simulink model "cyberAttack"  (R2022b)
settings: Solver=VariableStepAuto  StartTime=0.0  StopTime=10  RelTol=1e-3
values from neighbouring files (symbols this model uses):
  attackTimeDelay = 0.1    [editor.m]
  CC_Kd = 0    [editor.m]
  CC_Ki = 150    [editor.m]
  CC_Kp = 0    [editor.m]
  enableObserver = 1    [editor.m]
  ICapacity_1 = 3    [editor.m]
  ICapacity_2 = 2    [editor.m]
  ILoadFinal = 2    [editor.m]
  ILoadInitial = 3    [editor.m]
  Kd = 4.6e-4    (= 0.00046)    [editor.m]
  Ki = 6.15    [editor.m]
  Kp = 0.1    [editor.m]
  N = 2.56e3    (= 2560)    [editor.m]
  Rij = 0.05    [editor.m]
  Rt = 0.2    [editor.m]
  timeOfAttack = 5    [editor.m]
  tLoadChange = 6    [editor.m]
  Ts = 5e-5    (= 5e-05)    [editor.m]
  Vref = 40    [editor.m]
undefined symbols (not defined in the file or in its folder): Discrete, Time
libraries: fl_lib x27, nesl_utility_internal x15, slpidlib x4, simulink x2, ctrlSharedLib x2, ee_lib x2
(part 1 of 2)
settings Model: Creator=The MathWorks, Inc.  LastModifiedBy=bhuva

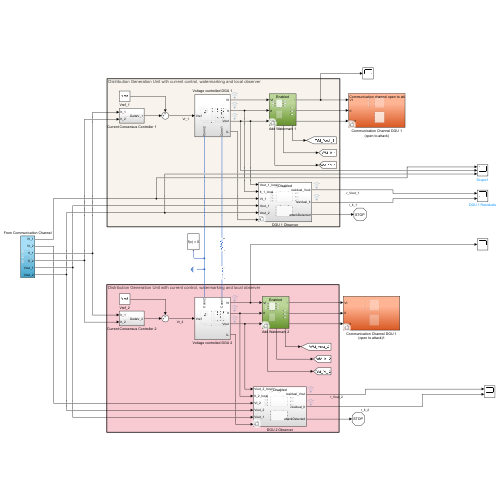
[thumbnail: Simulink's stored preview of the top-level diagram]
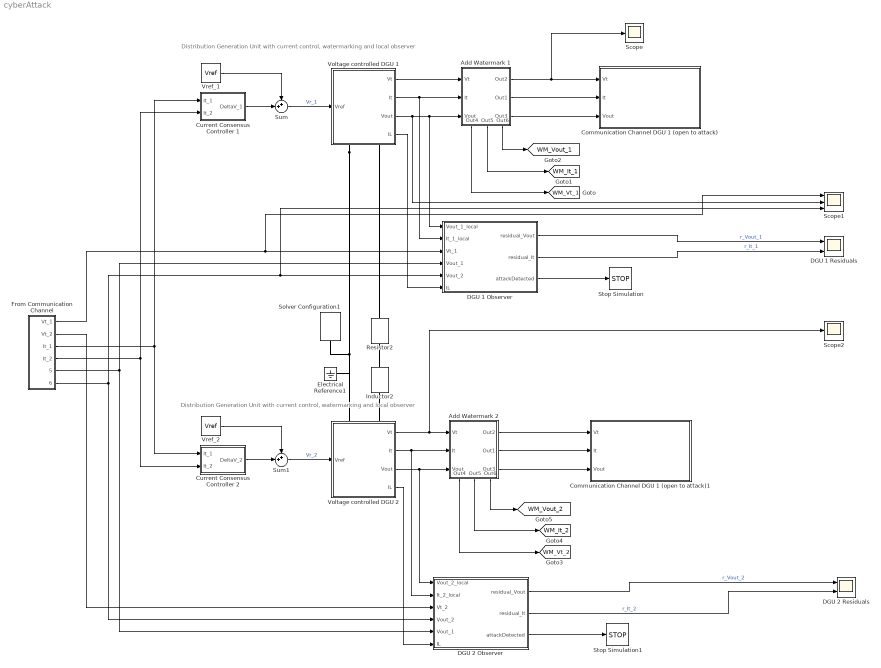
== system cyberAttack ==
  note: Distribution Generation Unit with current control, watermarking and local observer
  note: Distribution Generation Unit with current control, watermarking and local observer
  Add Watermark 1 : Subsystem  Variant=on  VariantControl=Choice
      settings: PortSchema="{\"entries\":[{\"content\":{\"sides\":[{\"content\":{\"connectorIds\":[\"In1\",\"In2\",\"In3\"]},\"type\":\"ConnectorPlacement.EquallySpacedRectSide\",\"uuid\":\"c94a7d77-0f2a-42c7-994c-f83d9f400b4a\"},{\"content\":{\"connectorIds\":[\"Out1\",\"Out2\",\"Out3\"],\"side\":\"RIGHT\"},\"type\":\"ConnectorPlacement.EquallySpacedRectSide\",\"uuid\":\"048bc904-366c-4deb-8d29-669922896a60\"},{\"content\":{\"connectorIds\":[],\"side\":\"TOP\"},\"type\":\"ConnectorPlacement.EquallySpacedRectSide\",\"uuid\":\"61856036-23df-49fc-9d48-72a95ac409b8\"},{\"content\":{\"connectorIds\":[\"Out4\",\"Out5\",\"Out6\"],\"side\":\"BOTTOM\"},\"type\":\"ConnectorPlacement.EquallySpacedRectSide\",\"uuid\":\"3c7882a6-545f-411e-a24e-2351be560f5c\"}]},\"type\":\"ConnectorPlacement.EquallySpacedConnector\",\"uuid\":\"82f313fb-6359-4167-9a1a-67611747de0f\"}],\"packageUris\":[\"http://schema.mathworks.com/mf0/Connector/R2020b\"],\"version\":\"1.0\"}"
  Add Watermark 2 : Subsystem  Variant=on  VariantControl=Choice
      settings: PortSchema="{\"entries\":[{\"content\":{\"sides\":[{\"content\":{\"connectorIds\":[\"In1\",\"In2\",\"In3\"]},\"type\":\"ConnectorPlacement.EquallySpacedRectSide\",\"uuid\":\"c94a7d77-0f2a-42c7-994c-f83d9f400b4a\"},{\"content\":{\"connectorIds\":[\"Out1\",\"Out2\",\"Out3\"],\"side\":\"RIGHT\"},\"type\":\"ConnectorPlacement.EquallySpacedRectSide\",\"uuid\":\"048bc904-366c-4deb-8d29-669922896a60\"},{\"content\":{\"connectorIds\":[],\"side\":\"TOP\"},\"type\":\"ConnectorPlacement.EquallySpacedRectSide\",\"uuid\":\"61856036-23df-49fc-9d48-72a95ac409b8\"},{\"content\":{\"connectorIds\":[\"Out4\",\"Out5\",\"Out6\"],\"side\":\"BOTTOM\"},\"type\":\"ConnectorPlacement.EquallySpacedRectSide\",\"uuid\":\"3c7882a6-545f-411e-a24e-2351be560f5c\"}]},\"type\":\"ConnectorPlacement.EquallySpacedConnector\",\"uuid\":\"82f313fb-6359-4167-9a1a-67611747de0f\"}],\"packageUris\":[\"http://schema.mathworks.com/mf0/Connector/R2020b\"],\"version\":\"1.0\"}"
  Communication Channel DGU 1 (open to attack) : Subsystem  Variant=on  VariantControl=Choice
  Communication Channel DGU 1 (open to attack)1 : Subsystem  Variant=on  VariantControl=Choice
  Current Consensus Controller 1 : Subsystem
  Current Consensus Controller 2 : Subsystem
  DGU 1 Observer : Subsystem  Variant=on  VariantControl=Choice
  DGU 1 Residuals : Scope  NumInputPorts=2
  DGU 2 Observer : Subsystem  Variant=on  VariantControl=Choice
  DGU 2 Residuals : Scope  NumInputPorts=2
  Electrical Reference1 : fl_lib/Electrical/Electrical Elements/Electrical Reference
  From Communication Channel : Subsystem
  Inductor2 : fl_lib/Electrical/Electrical Elements/Inductor  l=Lij H  r=0 Ohm  g=1e-9 1/Ohm  i_specify=off  i_priority=None  i=0 A  i_nominal_specify=off  i_nominal_unit=A  i_nominal_value=1  v_specify=off  v_priority=None  v=0 V  v_nominal_specify=off  v_nominal_unit=V  v_nominal_value=1  i_L_specify=off  i_L_priority=High  i_L=0 A  i_L_nominal_specify=off  i_L_nominal_unit=A  i_L_nominal_value=1
  Resistor2 : fl_lib/Electrical/Electrical Elements/Resistor  R=Rij Ohm  i_specify=off  i_priority=None  i=0 A  i_nominal_specify=off  i_nominal_unit=A  i_nominal_value=1  v_specify=off  v_priority=None  v=0 V  v_nominal_specify=off  v_nominal_unit=V  v_nominal_value=1
  Scope : Scope
  Scope1 : Scope  NumInputPorts=3
  Scope2 : Scope
  Solver Configuration1 : nesl_utility_internal/Solver Configuration  PhysicalDomain=network_engine_domain  SubClassName=solver  LeftPortType=input  RightPortType=generic  Tones=[]  Harmonics=[]  SimulateNoise=off  Profile=off  UseLocalSampling=off  EnableSwitchedLinearOptims=on  FrequencyDomain=off  UseCCode=off  RelTol=0.001  AbsTol=1e-06  MinStep=1e-09  ToWorkspace=off  RevertToSquareIcSolve=off  NumHomotopyIterations=100  PhasorMode=off  PhasorModeNumHarmonics=1  ConsistencySolver=NEWTON_FTOL  IndexReductionMethod=DerivativeReplacement  DoDC=off  ResidualTolerance=1e-9  ConsistencyTolSource=GLOBAL  ConsistencyAbsTol=0.001  ConsistencyRelTol=0.001  ConsistencyTolFactor=0.001  UseLocalSolver=on  LocalSolverChoice=NE_BACKWARD_EULER_ADVANCER  ResolveIndetEquations=on  FunctionEvalNumThread=1  LocalSolverSampleTime=Ts  DoFixedCost=on  MaxNonlinIter=3  MaxModeIter=2  ComputeImpulses=off  ImpulseIterations=2  LinearAlgebra=auto  LinearAlgebraNumThread=0  EquationFormulation=NE_TIME_EF  DelaysMemoryBudget=1024  AutomaticFiltering=on  FilteringTimeConstant=0.001  PartitionStorageMethod=AS_NEEDED  PartitionMemoryBudget=1024  PartitionMethod=FAST
  Stop Simulation : Stop
  Stop Simulation1 : Stop
  Sum : Sum  Inputs=++|
  Sum1 : Sum  Inputs=++|
  Voltage controlled DGU 1 : Subsystem
      settings: PortSchema="{\"entries\":[{\"content\":{\"sides\":[{\"content\":{\"connectorIds\":[]},\"type\":\"ConnectorPlacement.EquallySpacedRectSide\",\"uuid\":\"bd1f37b5-cace-475a-9319-df5dc175988c\"},{\"content\":{\"connectorIds\":[\"RConn1\",\"RConn2\"],\"side\":\"RIGHT\"},\"type\":\"ConnectorPlacement.EquallySpacedRectSide\",\"uuid\":\"6e9492d2-b492-4ddc-9bf9-c37fa50387fb\"},{\"content\":{\"connectorIds\":[\"Out1\",\"Out2\",\"Out3\",\"Out4\"],\"side\":\"TOP\"},\"type\":\"ConnectorPlacement.EquallySpacedRectSide\",\"uuid\":\"740d822e-a5fc-4d01-8f2e-7dd9c8c34700\"},{\"content\":{\"connectorIds\":[\"In1\"],\"side\":\"BOTTOM\"},\"type\":\"ConnectorPlacement.EquallySpacedRectSide\",\"uuid\":\"ce7350ec-18c7-472a-9669-30fb5abf65bf\"}]},\"type\":\"ConnectorPlacement.EquallySpacedConnector\",\"uuid\":\"15ef9329-fda5-41fa-bf9c-9b9fdaa2cf39\"}],\"packageUris\":[\"http://schema.mathworks.com/mf0/Connector/R2020b\"],\"version\":\"1.0\"}"
  Voltage controlled DGU 2 : Subsystem
      settings: PortSchema="{\"entries\":[{\"content\":{\"sides\":[{\"content\":{\"connectorIds\":[]},\"type\":\"ConnectorPlacement.EquallySpacedRectSide\",\"uuid\":\"bd1f37b5-cace-475a-9319-df5dc175988c\"},{\"content\":{\"connectorIds\":[\"RConn1\",\"RConn2\"],\"side\":\"RIGHT\"},\"type\":\"ConnectorPlacement.EquallySpacedRectSide\",\"uuid\":\"6e9492d2-b492-4ddc-9bf9-c37fa50387fb\"},{\"content\":{\"connectorIds\":[\"Out1\",\"Out2\",\"Out3\",\"Out4\"],\"side\":\"TOP\"},\"type\":\"ConnectorPlacement.EquallySpacedRectSide\",\"uuid\":\"740d822e-a5fc-4d01-8f2e-7dd9c8c34700\"},{\"content\":{\"connectorIds\":[\"In1\"],\"side\":\"BOTTOM\"},\"type\":\"ConnectorPlacement.EquallySpacedRectSide\",\"uuid\":\"ce7350ec-18c7-472a-9669-30fb5abf65bf\"}]},\"type\":\"ConnectorPlacement.EquallySpacedConnector\",\"uuid\":\"15ef9329-fda5-41fa-bf9c-9b9fdaa2cf39\"}],\"packageUris\":[\"http://schema.mathworks.com/mf0/Connector/R2020b\"],\"version\":\"1.0\"}"
  Vref_1 : Constant  Value=Vref  SampleTime=Ts
  Vref_2 : Constant  Value=Vref  SampleTime=Ts
  tag scope: WM_It_1=global, WM_It_2=global, WM_Vout_1=global, WM_Vout_2=global, WM_Vt_1=global, WM_Vt_2=global
  wires:
  Vref_1/1 -> Sum/1
  Sum/1 -> Voltage controlled DGU 1/1(Vref)  "Vr_1"
  Current Consensus Controller 1/1(DeltaV_1) -> Sum/2
  From Communication Channel/4(It_2) -> Current Consensus Controller 1/2(It_2), Current Consensus Controller 2/2(It_2)
  Voltage controlled DGU 1/3(Vout) -> Scope1/2, Add Watermark 1/3(Vout), DGU 1 Observer/1(Vout_1_local)
  Current Consensus Controller 2/1(DeltaV_2) -> Sum1/2
  Voltage controlled DGU 2/3(It) -> Add Watermark 2/2(It), DGU 2 Observer/2(It_2_local)
  Voltage controlled DGU 2/4(Vt) -> Scope2/1, Add Watermark 2/1(Vt)
  From Communication Channel/3(It_1) -> Current Consensus Controller 1/1(It_1), Current Consensus Controller 2/1(It_1)
  From Communication Channel/6(Vout_2) -> DGU 2 Observer/4(Vout_2), Scope1/3, DGU 1 Observer/5(Vout_2)
  Sum1/1 -> Voltage controlled DGU 2/1(Vref)  "Vr_2"
  From Communication Channel/5(Vout_1) -> DGU 2 Observer/5(Vout_1), DGU 1 Observer/4(Vout_1)
  Voltage controlled DGU 2/2(Vout) -> Add Watermark 2/3(Vout), DGU 2 Observer/1(Vout_2_local)
  Vref_2/1 -> Sum1/1
  Voltage controlled DGU 1/2(It) -> Add Watermark 1/2(It), DGU 1 Observer/2(It_1_local)
  DGU 2 Observer/3(attackDetected) -> Stop Simulation1/1
  From Communication Channel/1(Vt_1) -> Scope1/1, DGU 1 Observer/3(Vt_1)
  Voltage controlled DGU 1/4(IL) -> DGU 1 Observer/6(IL)
  From Communication Channel/2(Vt_2) -> DGU 2 Observer/3(Vt_2)
  Voltage controlled DGU 1/1(Vt) -> Add Watermark 1/1(Vt)
  Add Watermark 1/1(Out2) -> Scope/1, Communication Channel DGU 1 (open to attack)/1(Vt)
  Add Watermark 1/2(Out1) -> Communication Channel DGU 1 (open to attack)/2(It)
  Add Watermark 1/3(Out3) -> Communication Channel DGU 1 (open to attack)/3(Vout)
  Add Watermark 1/4(Out4) -> [WM_Vt_1]
  Add Watermark 1/5(Out5) -> [WM_It_1]
  Add Watermark 1/6(Out6) -> [WM_Vout_1]
  DGU 1 Observer/1(residual_Vout) -> DGU 1 Residuals/1  "r_Vout_1"
  DGU 1 Observer/2(residual_It) -> DGU 1 Residuals/2  "r_It_1"
  DGU 1 Observer/3(attackDetected) -> Stop Simulation/1
  Voltage controlled DGU 2/1(IL) -> DGU 2 Observer/6(IL)
  DGU 2 Observer/1(residual_Vout) -> DGU 2 Residuals/1  "r_Vout_2"
  DGU 2 Observer/2(residual_It) -> DGU 2 Residuals/2  "r_It_2"
  Add Watermark 2/6(Out6) -> [WM_Vout_2]
  Add Watermark 2/5(Out5) -> [WM_It_2]
  Add Watermark 2/4(Out4) -> [WM_Vt_2]
  Add Watermark 2/1(Out2) -> Communication Channel DGU 1 (open to attack)1/1(Vt)
  Add Watermark 2/2(Out1) -> Communication Channel DGU 1 (open to attack)1/2(It)
  Add Watermark 2/3(Out3) -> Communication Channel DGU 1 (open to attack)1/3(Vout)
  connections:
  Voltage controlled DGU 1/RConn2 -- Electrical Reference1/LConn1 -- Voltage controlled DGU 2/RConn2 -- Solver Configuration1/RConn1
  Inductor2/LConn1 -- Resistor2/RConn1
  Voltage controlled DGU 2/RConn1 -- Inductor2/RConn1
  Resistor2/LConn1 -- Voltage controlled DGU 1/RConn1

== system cyberAttack/Add Watermark 1 ==
  Vt : Inport
  It : Inport  Port=2
  Vout : Inport  Port=3
  Disabled : Subsystem  VariantControl=enableWatermarking == 0
      settings: PortSchema="{\"entries\":[{\"content\":{\"sides\":[{\"content\":{\"connectorIds\":[\"In1\",\"In2\",\"In3\"]},\"type\":\"ConnectorPlacement.EquallySpacedRectSide\",\"uuid\":\"c94a7d77-0f2a-42c7-994c-f83d9f400b4a\"},{\"content\":{\"connectorIds\":[\"Out1\",\"Out2\",\"Out3\"],\"side\":\"RIGHT\"},\"type\":\"ConnectorPlacement.EquallySpacedRectSide\",\"uuid\":\"048bc904-366c-4deb-8d29-669922896a60\"},{\"content\":{\"connectorIds\":[],\"side\":\"TOP\"},\"type\":\"ConnectorPlacement.EquallySpacedRectSide\",\"uuid\":\"61856036-23df-49fc-9d48-72a95ac409b8\"},{\"content\":{\"connectorIds\":[\"Out4\",\"Out5\",\"Out6\"],\"side\":\"BOTTOM\"},\"type\":\"ConnectorPlacement.EquallySpacedRectSide\",\"uuid\":\"3c7882a6-545f-411e-a24e-2351be560f5c\"}]},\"type\":\"ConnectorPlacement.EquallySpacedConnector\",\"uuid\":\"82f313fb-6359-4167-9a1a-67611747de0f\"}],\"packageUris\":[\"http://schema.mathworks.com/mf0/Connector/R2020b\"],\"version\":\"1.0\"}"
  Enabled : Subsystem  VariantControl=enableWatermarking == 1
      settings: PortSchema="{\"entries\":[{\"content\":{\"sides\":[{\"content\":{\"connectorIds\":[\"In1\",\"In2\",\"In3\"]},\"type\":\"ConnectorPlacement.EquallySpacedRectSide\",\"uuid\":\"c94a7d77-0f2a-42c7-994c-f83d9f400b4a\"},{\"content\":{\"connectorIds\":[\"Out1\",\"Out2\",\"Out3\"],\"side\":\"RIGHT\"},\"type\":\"ConnectorPlacement.EquallySpacedRectSide\",\"uuid\":\"048bc904-366c-4deb-8d29-669922896a60\"},{\"content\":{\"connectorIds\":[],\"side\":\"TOP\"},\"type\":\"ConnectorPlacement.EquallySpacedRectSide\",\"uuid\":\"61856036-23df-49fc-9d48-72a95ac409b8\"},{\"content\":{\"connectorIds\":[\"Out4\",\"Out5\",\"Out6\"],\"side\":\"BOTTOM\"},\"type\":\"ConnectorPlacement.EquallySpacedRectSide\",\"uuid\":\"3c7882a6-545f-411e-a24e-2351be560f5c\"}]},\"type\":\"ConnectorPlacement.EquallySpacedConnector\",\"uuid\":\"82f313fb-6359-4167-9a1a-67611747de0f\"}],\"packageUris\":[\"http://schema.mathworks.com/mf0/Connector/R2020b\"],\"version\":\"1.0\"}"
  Out2 : Outport
  Out1 : Outport  Port=2
  Out3 : Outport  Port=3
  Out4 : Outport  Port=4
  Out5 : Outport  Port=5
  Out6 : Outport  Port=6

== system cyberAttack/Add Watermark 2 ==
  Vt : Inport
  It : Inport  Port=2
  Vout : Inport  Port=3
  Disabled : Subsystem  VariantControl=enableWatermarking == 0
      settings: PortSchema="{\"entries\":[{\"content\":{\"sides\":[{\"content\":{\"connectorIds\":[\"In1\",\"In2\",\"In3\"]},\"type\":\"ConnectorPlacement.EquallySpacedRectSide\",\"uuid\":\"c94a7d77-0f2a-42c7-994c-f83d9f400b4a\"},{\"content\":{\"connectorIds\":[\"Out1\",\"Out2\",\"Out3\"],\"side\":\"RIGHT\"},\"type\":\"ConnectorPlacement.EquallySpacedRectSide\",\"uuid\":\"048bc904-366c-4deb-8d29-669922896a60\"},{\"content\":{\"connectorIds\":[],\"side\":\"TOP\"},\"type\":\"ConnectorPlacement.EquallySpacedRectSide\",\"uuid\":\"61856036-23df-49fc-9d48-72a95ac409b8\"},{\"content\":{\"connectorIds\":[\"Out4\",\"Out5\",\"Out6\"],\"side\":\"BOTTOM\"},\"type\":\"ConnectorPlacement.EquallySpacedRectSide\",\"uuid\":\"3c7882a6-545f-411e-a24e-2351be560f5c\"}]},\"type\":\"ConnectorPlacement.EquallySpacedConnector\",\"uuid\":\"82f313fb-6359-4167-9a1a-67611747de0f\"}],\"packageUris\":[\"http://schema.mathworks.com/mf0/Connector/R2020b\"],\"version\":\"1.0\"}"
  Enabled : Subsystem  VariantControl=enableWatermarking == 1
      settings: PortSchema="{\"entries\":[{\"content\":{\"sides\":[{\"content\":{\"connectorIds\":[\"In1\",\"In2\",\"In3\"]},\"type\":\"ConnectorPlacement.EquallySpacedRectSide\",\"uuid\":\"c94a7d77-0f2a-42c7-994c-f83d9f400b4a\"},{\"content\":{\"connectorIds\":[\"Out1\",\"Out2\",\"Out3\"],\"side\":\"RIGHT\"},\"type\":\"ConnectorPlacement.EquallySpacedRectSide\",\"uuid\":\"048bc904-366c-4deb-8d29-669922896a60\"},{\"content\":{\"connectorIds\":[],\"side\":\"TOP\"},\"type\":\"ConnectorPlacement.EquallySpacedRectSide\",\"uuid\":\"61856036-23df-49fc-9d48-72a95ac409b8\"},{\"content\":{\"connectorIds\":[\"Out4\",\"Out5\",\"Out6\"],\"side\":\"BOTTOM\"},\"type\":\"ConnectorPlacement.EquallySpacedRectSide\",\"uuid\":\"3c7882a6-545f-411e-a24e-2351be560f5c\"}]},\"type\":\"ConnectorPlacement.EquallySpacedConnector\",\"uuid\":\"82f313fb-6359-4167-9a1a-67611747de0f\"}],\"packageUris\":[\"http://schema.mathworks.com/mf0/Connector/R2020b\"],\"version\":\"1.0\"}"
  Out2 : Outport
  Out1 : Outport  Port=2
  Out3 : Outport  Port=3
  Out4 : Outport  Port=4
  Out5 : Outport  Port=5
  Out6 : Outport  Port=6

== system cyberAttack/Communication Channel DGU 1 (open to attack) ==
  Vt : Inport
  It : Inport  Port=2
  Vout : Inport  Port=3
  Communication Channel : Subsystem  VariantControl=enableAttack == 0
  Communication channel open to attack : Subsystem  VariantControl=enableAttack == 1

== system cyberAttack/Communication Channel DGU 1 (open to attack)1 ==
  Vt : Inport
  It : Inport  Port=2
  Vout : Inport  Port=3
  Communication Channel : Subsystem  VariantControl=enableAttack1 == 0
  Communication channel open to attack : Subsystem  VariantControl=enableAttack1 == 1

== system cyberAttack/Current Consensus Controller 1 ==
  It_1 : Inport
  It_2 : Inport  Port=2
  Discrete PID Controller : slpidlib/PID Controller  Controller=PID  Form=Parallel  TimeDomain=Discrete-time  UseExternalTs=off  SampleTime=Ts  IntegratorMethod=Forward Euler  FilterMethod=Forward Euler  ControllerParametersSource=internal  P=CC_Kp  I=CC_Ki  UseKiTs=off  D=CC_Kd  N=1e4  UseFilter=on  TunerSelectOption=Transfer Function Based (PID Tuner App)  InitialConditionSource=internal  InitialConditionForIntegrator=0  InitialConditionForFilter=0  DifferentiatorICPrevScaledInput=0  ExternalReset=none  TrackingMode=off  Kt=1  LimitOutput=off  SatLimitsSource=internal  UpperSaturationLimit=inf  LowerSaturationLimit=-inf  LinearizeAsGain=off  AntiWindupMode=none  Kb=1  LimitIntegrator=off  UpperIntegratorSaturationLimit=inf  LowerIntegratorSaturationLimit=-inf  POutMin=[]  POutMax=[]  IOutMin=[]  IOutMax=[]  DOutMin=[]  DOutMax=[]  NOutMin=[]  NOutMax=[]  SumOutMin=[]  SumOutMax=[]  SaturationOutMin=[]  SaturationOutMax=[]  PParamMin=[]  PParamMax=[]  IParamMin=[]  IParamMax=[]  DParamMin=[]  DParamMax=[]  NParamMin=[]  NParamMax=[]  KbParamMin=[]  KbParamMax=[]  KtParamMin=[]  KtParamMax=[]  KbOutMin=[]  KbOutMax=[]  KtOutMin=[]  KtOutMax=[]  IntegratorOutMin=[]  IntegratorOutMax=[]  FilterOutMin=[]  FilterOutMax=[]  SumI1OutMin=[]  SumI1OutMax=[]  SumI2OutMin=[]  SumI2OutMax=[]  SumI3OutMin=[]  SumI3OutMax=[]  SumI4OutMin=[]  SumI4OutMax=[]  SumDOutMin=[]  SumDOutMax=[]  DifferentiatorOutMin=[]  DifferentiatorOutMax=[]  FilterDiffOutCoefMin=[]  FilterDiffOutCoefMax=[]  ReciprocalOutMin=[]  ReciprocalOutMax=[]  SumDenOutMin=[]  SumDenOutMax=[]  SumNumOutMin=[]  SumNumOutMax=[]  DivideOutMin=[]  DivideOutMax=[]  UdiffTsProdOutMin=[]  UdiffTsProdOutMax=[]  NTsProdOutMin=[]  NTsProdOutMax=[]  UintegralTsProdOutMin=[]  UintegralTsProdOutMax=[]  UngainTsProdOutMin=[]  UngainTsProdOutMax=[]  ClampingZeroOutDataTypeStr=Inherit: Inherit via back propagation  ClampingZeroOutMin=[]  ClampingZeroOutMax=[]  FilterDenConstantOutDataTypeStr=Inherit: Inherit via back propagation  FilterDenConstantOutMin=[]  FilterDenConstantOutMax=[]  PCopyOutDataTypeStr=Inherit: Inherit via back propagation  PCopyOutMin=[]  PCopyOutMax=[]  NCopyOutDataTypeStr=Inherit: Inherit via back propagation  NCopyOutMin=[]  NCopyOutMax=[]  IntegratorContinuousStateAttributes=''  IntegratorStateMustResolveToSignalObject=off  IntegratorRTWStateStorageClass=Auto  FilterContinuousStateAttributes=''  FilterStateMustResolveToSignalObject=off  FilterRTWStateStorageClass=Auto  ParallelPVariant=InternalParameters  IdealPVariant=Disabled  IVariant=InternalParameters  DVariant=InternalParameters  IntegratorVariant=Discrete  SatVariant=Disabled  AWVariant=Passthrough  PCopyVariant=Disabled  TRVariant=Disabled  FdbkBlocksVariant=Forward  IdealPFdbkVariant=Disabled  SatFdbkVariant=Disabled  DerivativeFilterVariant=ForwardEulerFilter  NVariant=InternalParameters  NCopyVariant=Disabled  FilterICVariant=InternalICsFilter  IntegratorICVariant=InternalICs  ExternalResetVariant=Disabled  TRSumVariant=Passthrough  SumFdbkVariant=Disabled  SumVariant=Sum_PID  TsampFilterVariant=InternalTs  TsampNgainVariant=Passthrough  TsampIntegralVariant=Passthrough  ExternalSaturationOutDataTypeStr=Inherit: Same as second input
      settings: LibrarySourceBlock=simulink/Discrete/Discrete PID Controller
  Gain7 : Gain  Gain=1/ICapacity_1
  Gain8 : Gain  Gain=1/ICapacity_2
  Sum : Sum  Inputs=-+|
  Sum1 : Sum  Inputs=-+|
  Sum4 : Sum  Inputs=|-+
  DeltaV_1 : Outport
  wires:
  Gain8/1 -> Sum4/2
  It_2/1 -> Sum1/2
  Gain7/1 -> Sum4/1
  Discrete PID Controller/1 -> DeltaV_1/1
  Sum/1 -> Gain7/1
  Sum1/1 -> Gain8/1
  It_1/1 -> Sum/2
  [WM_It_1] -> Sum/1
  [WM_It_2] -> Sum1/1
  Sum4/1 -> Discrete PID Controller/1

== system cyberAttack/Current Consensus Controller 2 ==
  It_1 : Inport
  It_2 : Inport  Port=2
  Discrete PID Controller : slpidlib/PID Controller  Controller=PID  Form=Parallel  TimeDomain=Discrete-time  UseExternalTs=off  SampleTime=Ts  IntegratorMethod=Forward Euler  FilterMethod=Forward Euler  ControllerParametersSource=internal  P=CC_Kp  I=CC_Ki  UseKiTs=off  D=CC_Kd  N=1e4  UseFilter=on  TunerSelectOption=Transfer Function Based (PID Tuner App)  InitialConditionSource=internal  InitialConditionForIntegrator=0  InitialConditionForFilter=0  DifferentiatorICPrevScaledInput=0  ExternalReset=none  TrackingMode=off  Kt=1  LimitOutput=off  SatLimitsSource=internal  UpperSaturationLimit=inf  LowerSaturationLimit=-inf  LinearizeAsGain=off  AntiWindupMode=none  Kb=1  LimitIntegrator=off  UpperIntegratorSaturationLimit=inf  LowerIntegratorSaturationLimit=-inf  POutMin=[]  POutMax=[]  IOutMin=[]  IOutMax=[]  DOutMin=[]  DOutMax=[]  NOutMin=[]  NOutMax=[]  SumOutMin=[]  SumOutMax=[]  SaturationOutMin=[]  SaturationOutMax=[]  PParamMin=[]  PParamMax=[]  IParamMin=[]  IParamMax=[]  DParamMin=[]  DParamMax=[]  NParamMin=[]  NParamMax=[]  KbParamMin=[]  KbParamMax=[]  KtParamMin=[]  KtParamMax=[]  KbOutMin=[]  KbOutMax=[]  KtOutMin=[]  KtOutMax=[]  IntegratorOutMin=[]  IntegratorOutMax=[]  FilterOutMin=[]  FilterOutMax=[]  SumI1OutMin=[]  SumI1OutMax=[]  SumI2OutMin=[]  SumI2OutMax=[]  SumI3OutMin=[]  SumI3OutMax=[]  SumI4OutMin=[]  SumI4OutMax=[]  SumDOutMin=[]  SumDOutMax=[]  DifferentiatorOutMin=[]  DifferentiatorOutMax=[]  FilterDiffOutCoefMin=[]  FilterDiffOutCoefMax=[]  ReciprocalOutMin=[]  ReciprocalOutMax=[]  SumDenOutMin=[]  SumDenOutMax=[]  SumNumOutMin=[]  SumNumOutMax=[]  DivideOutMin=[]  DivideOutMax=[]  UdiffTsProdOutMin=[]  UdiffTsProdOutMax=[]  NTsProdOutMin=[]  NTsProdOutMax=[]  UintegralTsProdOutMin=[]  UintegralTsProdOutMax=[]  UngainTsProdOutMin=[]  UngainTsProdOutMax=[]  ClampingZeroOutDataTypeStr=Inherit: Inherit via back propagation  ClampingZeroOutMin=[]  ClampingZeroOutMax=[]  FilterDenConstantOutDataTypeStr=Inherit: Inherit via back propagation  FilterDenConstantOutMin=[]  FilterDenConstantOutMax=[]  PCopyOutDataTypeStr=Inherit: Inherit via back propagation  PCopyOutMin=[]  PCopyOutMax=[]  NCopyOutDataTypeStr=Inherit: Inherit via back propagation  NCopyOutMin=[]  NCopyOutMax=[]  IntegratorContinuousStateAttributes=''  IntegratorStateMustResolveToSignalObject=off  IntegratorRTWStateStorageClass=Auto  FilterContinuousStateAttributes=''  FilterStateMustResolveToSignalObject=off  FilterRTWStateStorageClass=Auto  ParallelPVariant=InternalParameters  IdealPVariant=Disabled  IVariant=InternalParameters  DVariant=InternalParameters  IntegratorVariant=Discrete  SatVariant=Disabled  AWVariant=Passthrough  PCopyVariant=Disabled  TRVariant=Disabled  FdbkBlocksVariant=Forward  IdealPFdbkVariant=Disabled  SatFdbkVariant=Disabled  DerivativeFilterVariant=ForwardEulerFilter  NVariant=InternalParameters  NCopyVariant=Disabled  FilterICVariant=InternalICsFilter  IntegratorICVariant=InternalICs  ExternalResetVariant=Disabled  TRSumVariant=Passthrough  SumFdbkVariant=Disabled  SumVariant=Sum_PID  TsampFilterVariant=InternalTs  TsampNgainVariant=Passthrough  TsampIntegralVariant=Passthrough  ExternalSaturationOutDataTypeStr=Inherit: Same as second input
      settings: LibrarySourceBlock=simulink/Discrete/Discrete PID Controller
  Gain7 : Gain  Gain=1/ICapacity_1
  Gain8 : Gain  Gain=1/ICapacity_2
  Sum : Sum  Inputs=-+|
  Sum1 : Sum  Inputs=-+|
  Sum4 : Sum  Inputs=|+-
  DeltaV_2 : Outport
  wires:
  Gain8/1 -> Sum4/2
  It_2/1 -> Sum1/2
  Sum4/1 -> Discrete PID Controller/1
  Gain7/1 -> Sum4/1
  Discrete PID Controller/1 -> DeltaV_2/1
  Sum/1 -> Gain7/1
  Sum1/1 -> Gain8/1
  It_1/1 -> Sum/2
  [WM_It_1] -> Sum/1
  [WM_It_2] -> Sum1/1

== system cyberAttack/DGU 1 Observer ==
  Vout_1_local : Inport
  It_1_local : Inport  Port=2
  Vt_1 : Inport  Port=3
  Vout_1 : Inport  Port=4
  Vout_2 : Inport  Port=5
  IL : Inport  Port=6
  Disabled : Subsystem  VariantControl=enableObserver == 0
      settings: PortSchema="{\"entries\":[{\"content\":{\"sides\":[{\"content\":{\"connectorIds\":[\"In1\",\"In2\",\"In3\",\"In4\"]},\"type\":\"ConnectorPlacement.EquallySpacedRectSide\",\"uuid\":\"1fcbc3c4-c380-448d-a7a8-357aa057b5ad\"},{\"content\":{\"connectorIds\":[\"Out1\",\"Out2\",\"Out3\"],\"side\":\"RIGHT\"},\"type\":\"ConnectorPlacement.EquallySpacedRectSide\",\"uuid\":\"7cbaad62-7890-4094-8ace-3159eca04825\"},{\"content\":{\"connectorIds\":[\"In5\",\"In6\"],\"side\":\"TOP\"},\"type\":\"ConnectorPlacement.EquallySpacedRectSide\",\"uuid\":\"f6c34017-9df2-4479-96e0-d67eb53c1d2d\"}]},\"type\":\"ConnectorPlacement.EquallySpacedConnector\",\"uuid\":\"f0a4a9b8-ed06-4c65-915f-6b202d377626\"}],\"packageUris\":[\"http://schema.mathworks.com/mf0/Connector/R2020b\"],\"version\":\"1.0\"}"
  Enabled : Subsystem  VariantControl=enableObserver == 1
      settings: PortSchema="{\"entries\":[{\"content\":{\"sides\":[{\"content\":{\"connectorIds\":[\"In1\",\"In2\",\"In3\",\"In4\"]},\"type\":\"ConnectorPlacement.EquallySpacedRectSide\",\"uuid\":\"1fcbc3c4-c380-448d-a7a8-357aa057b5ad\"},{\"content\":{\"connectorIds\":[\"Out1\",\"Out2\",\"Out3\"],\"side\":\"RIGHT\"},\"type\":\"ConnectorPlacement.EquallySpacedRectSide\",\"uuid\":\"7cbaad62-7890-4094-8ace-3159eca04825\"},{\"content\":{\"connectorIds\":[\"In5\",\"In6\"],\"side\":\"TOP\"},\"type\":\"ConnectorPlacement.EquallySpacedRectSide\",\"uuid\":\"f6c34017-9df2-4479-96e0-d67eb53c1d2d\"}]},\"type\":\"ConnectorPlacement.EquallySpacedConnector\",\"uuid\":\"f0a4a9b8-ed06-4c65-915f-6b202d377626\"}],\"packageUris\":[\"http://schema.mathworks.com/mf0/Connector/R2020b\"],\"version\":\"1.0\"}"
  residual_Vout : Outport
  residual_It : Outport  Port=2
  attackDetected : Outport  Port=3

== system cyberAttack/DGU 2 Observer ==
  Vout_2_local : Inport
  It_2_local : Inport  Port=2
  Vt_2 : Inport  Port=3
  Vout_2 : Inport  Port=4
  Vout_1 : Inport  Port=5
  IL : Inport  Port=6
  Disabled : Subsystem  VariantControl=enableObserver == 0
      settings: PortSchema="{\"entries\":[{\"content\":{\"sides\":[{\"content\":{\"connectorIds\":[\"In1\",\"In2\",\"In3\",\"In4\"]},\"type\":\"ConnectorPlacement.EquallySpacedRectSide\",\"uuid\":\"1fcbc3c4-c380-448d-a7a8-357aa057b5ad\"},{\"content\":{\"connectorIds\":[\"Out1\",\"Out2\",\"Out3\"],\"side\":\"RIGHT\"},\"type\":\"ConnectorPlacement.EquallySpacedRectSide\",\"uuid\":\"7cbaad62-7890-4094-8ace-3159eca04825\"},{\"content\":{\"connectorIds\":[\"In5\",\"In6\"],\"side\":\"TOP\"},\"type\":\"ConnectorPlacement.EquallySpacedRectSide\",\"uuid\":\"f6c34017-9df2-4479-96e0-d67eb53c1d2d\"}]},\"type\":\"ConnectorPlacement.EquallySpacedConnector\",\"uuid\":\"f0a4a9b8-ed06-4c65-915f-6b202d377626\"}],\"packageUris\":[\"http://schema.mathworks.com/mf0/Connector/R2020b\"],\"version\":\"1.0\"}"
  Enabled : Subsystem  VariantControl=enableObserver == 1
      settings: PortSchema="{\"entries\":[{\"content\":{\"sides\":[{\"content\":{\"connectorIds\":[\"In1\",\"In2\",\"In3\",\"In4\"]},\"type\":\"ConnectorPlacement.EquallySpacedRectSide\",\"uuid\":\"1fcbc3c4-c380-448d-a7a8-357aa057b5ad\"},{\"content\":{\"connectorIds\":[\"Out1\",\"Out2\",\"Out3\"],\"side\":\"RIGHT\"},\"type\":\"ConnectorPlacement.EquallySpacedRectSide\",\"uuid\":\"7cbaad62-7890-4094-8ace-3159eca04825\"},{\"content\":{\"connectorIds\":[\"In5\",\"In6\"],\"side\":\"TOP\"},\"type\":\"ConnectorPlacement.EquallySpacedRectSide\",\"uuid\":\"f6c34017-9df2-4479-96e0-d67eb53c1d2d\"}]},\"type\":\"ConnectorPlacement.EquallySpacedConnector\",\"uuid\":\"f0a4a9b8-ed06-4c65-915f-6b202d377626\"}],\"packageUris\":[\"http://schema.mathworks.com/mf0/Connector/R2020b\"],\"version\":\"1.0\"}"
  residual_Vout : Outport
  residual_It : Outport  Port=2
  attackDetected : Outport  Port=3

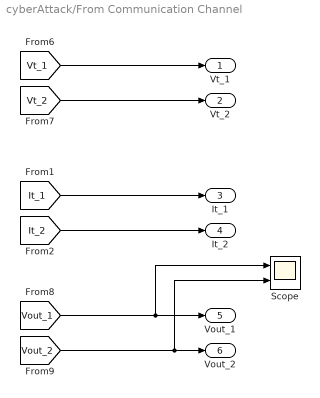
== system cyberAttack/From Communication Channel ==
  Scope : Scope  NumInputPorts=2
  Vt_1 : Outport
  Vt_2 : Outport  Port=2
  It_1 : Outport  Port=3
  It_2 : Outport  Port=4
  Vout_1 : Outport  Port=5
  Vout_2 : Outport  Port=6
  wires:
  [Vout_2] -> Scope/2, Vout_2/1
  [Vt_1] -> Vt_1/1
  [It_1] -> It_1/1
  [Vout_1] -> Scope/1, Vout_1/1
  [Vt_2] -> Vt_2/1
  [It_2] -> It_2/1

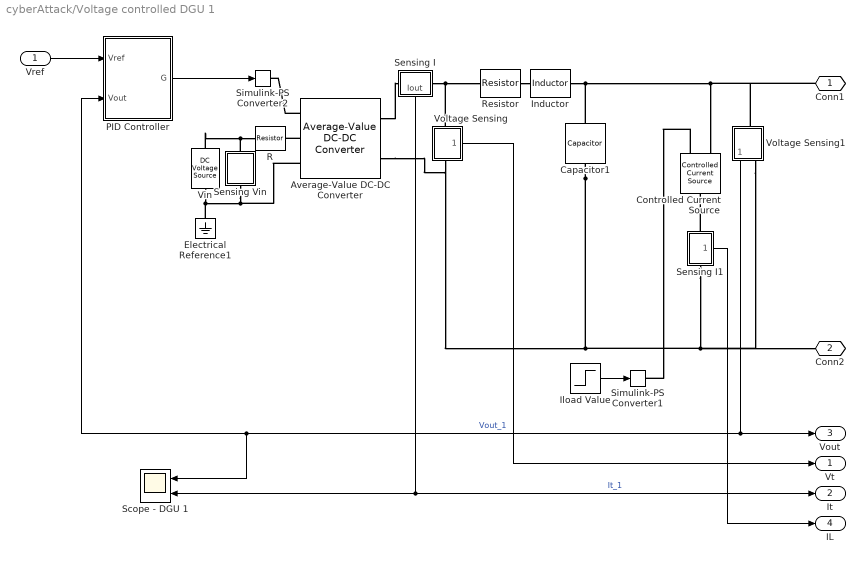
== system cyberAttack/Voltage controlled DGU 1 ==
  Vref : Inport
  Average-Value DC-DC Converter : ee_lib/Semiconductors & Converters/Converters/Average-Value DC-DC Converter  control_option=ee.enum.converters.controlinput.dutycycle  converter_type=ee.enum.converters.dcdctype.buck  efficiency_option=ee.enum.converters.efficiency.constant  efficiency_fixed=100  i_vec=[0, 2, 5] A  efficiency_vec=[90, 95, 98]
      settings: InternalSimscapePortConfiguration="{\"Bottom\":[],\"Left\":[{\"id\":\"DutyCycle\",\"label\":\"DutyCycle\",\"type\":\"input\"},{\"id\":\"p1\",\"label\":\"1+\",\"type\":\"foundation.electrical.electrical\"},{\"id\":\"n1\",\"label\":\"1-\",\"type\":\"foundation.electrical.electrical\"}],\"Right\":[{\"id\":\"p2\",\"label\":\"2+\",\"type\":\"foundation.electrical.electrical\"},{\"id\":\"n2\",\"label\":\"2-\",\"type\":\"foundation.electrical.electrical\"}],\"Top\":[]}"
  Capacitor1 : fl_lib/Electrical/Electrical Elements/Capacitor  c=Ct F  r=1e-6 Ohm  g=0 1/Ohm  i_specify=off  i_priority=None  i=0 A  i_nominal_specify=off  i_nominal_unit=A  i_nominal_value=1  v_specify=on  v_priority=None  v=80 V  v_nominal_specify=off  v_nominal_unit=V  v_nominal_value=1  vc_specify=off  vc_priority=High  vc=0 V  vc_nominal_specify=off  vc_nominal_unit=V  vc_nominal_value=1
  Controlled Current Source : fl_lib/Electrical/Electrical Sources/Controlled Current Source
  Electrical Reference1 : fl_lib/Electrical/Electrical Elements/Electrical Reference
  Iload Value : Step  Time=tLoadChange  Before=ILoadInitial  After=ILoadFinal  SampleTime=Ts  VectorParams1D=off
  Inductor : fl_lib/Electrical/Electrical Elements/Inductor  l=Lt H  r=0 Ohm  g=1e-9 1/Ohm  i_specify=off  i_priority=None  i=0 A  i_nominal_specify=off  i_nominal_unit=A  i_nominal_value=1  v_specify=off  v_priority=None  v=0 V  v_nominal_specify=off  v_nominal_unit=V  v_nominal_value=1  i_L_specify=off  i_L_priority=High  i_L=0 A  i_L_nominal_specify=off  i_L_nominal_unit=A  i_L_nominal_value=1
  PID Controller : Subsystem  VariantControl=PID Controller
  R : fl_lib/Electrical/Electrical Elements/Resistor  R=0.001 Ohm  i_specify=off  i_priority=None  i=0 A  i_nominal_specify=off  i_nominal_unit=A  i_nominal_value=1  v_specify=off  v_priority=None  v=0 V  v_nominal_specify=off  v_nominal_unit=V  v_nominal_value=1
  Resistor : fl_lib/Electrical/Electrical Elements/Resistor  R=Rt Ohm  i_specify=off  i_priority=None  i=0 A  i_nominal_specify=off  i_nominal_unit=A  i_nominal_value=1  v_specify=off  v_priority=None  v=0 V  v_nominal_specify=off  v_nominal_unit=V  v_nominal_value=1
  Scope - DGU 1 : Scope  NumInputPorts=2
  Sensing Vin : Subsystem
      mask Display:
      | disp('V')
      | port_label('Lconn',1,'+')
      | port_label('Rconn',1,'-')
  Sensing I : Subsystem
      settings: PortSchema="{\"entries\":[{\"content\":{\"sides\":[{\"content\":{\"connectorIds\":[\"LConn1\"]},\"type\":\"ConnectorPlacement.EquallySpacedRectSide\",\"uuid\":\"8998040f-d19b-40f6-852f-9dc0afd5a871\"},{\"content\":{\"connectorIds\":[\"RConn1\"],\"side\":\"RIGHT\"},\"type\":\"ConnectorPlacement.EquallySpacedRectSide\",\"uuid\":\"65494d6e-d653-4050-90f0-55ab431a5ea5\"},{\"content\":{\"connectorIds\":[],\"side\":\"TOP\"},\"type\":\"ConnectorPlacement.EquallySpacedRectSide\",\"uuid\":\"2b796c8d-afa9-4f67-a302-9fd74e5c5a87\"},{\"content\":{\"connectorIds\":[\"Out1\"],\"side\":\"BOTTOM\"},\"type\":\"ConnectorPlacement.EquallySpacedRectSide\",\"uuid\":\"a59db07b-fad7-4423-9f0d-248c8e243318\"}]},\"type\":\"ConnectorPlacement.EquallySpacedConnector\",\"uuid\":\"55bdfac7-fde1-4547-95b0-f675ec2b07db\"}],\"packageUris\":[\"http://schema.mathworks.com/mf0/Connector/R2020b\"],\"version\":\"1.0\"}"
      mask Display:
      | disp('I')
      | port_label('Lconn',1,'+')
      | port_label('Rconn',1,'-')
  Sensing I1 : Subsystem
      settings: PortSchema="{\"entries\":[{\"content\":{\"sides\":[{\"content\":{\"connectorIds\":[\"LConn1\"]},\"type\":\"ConnectorPlacement.EquallySpacedRectSide\",\"uuid\":\"8998040f-d19b-40f6-852f-9dc0afd5a871\"},{\"content\":{\"connectorIds\":[\"RConn1\"],\"side\":\"RIGHT\"},\"type\":\"ConnectorPlacement.EquallySpacedRectSide\",\"uuid\":\"65494d6e-d653-4050-90f0-55ab431a5ea5\"},{\"content\":{\"connectorIds\":[\"Out1\"],\"side\":\"TOP\"},\"type\":\"ConnectorPlacement.EquallySpacedRectSide\",\"uuid\":\"2b796c8d-afa9-4f67-a302-9fd74e5c5a87\"},{\"content\":{\"connectorIds\":[],\"side\":\"BOTTOM\"},\"type\":\"ConnectorPlacement.EquallySpacedRectSide\",\"uuid\":\"a59db07b-fad7-4423-9f0d-248c8e243318\"}]},\"type\":\"ConnectorPlacement.EquallySpacedConnector\",\"uuid\":\"55bdfac7-fde1-4547-95b0-f675ec2b07db\"}],\"packageUris\":[\"http://schema.mathworks.com/mf0/Connector/R2020b\"],\"version\":\"1.0\"}"
      mask Display:
      | disp('I')
      | port_label('Lconn',1,'+')
      | port_label('Rconn',1,'-')
  Simulink-PS Converter1 : nesl_utility_internal/Simulink-PS Converter  PhysicalDomain=network_engine_domain  SubClassName=ps_input  LeftPortType=input  RightPortType=output  PseudoPeriodic=off  Frequencies=[]  NoiseDistribution=none  NoiseParameters=[]  Unit=1  AffineConversion=off  FilteringAndDerivatives=zero  SimscapeFilterOrder=1  InputFilterTimeConstant=0.001  UdotUserProvided=0
  Simulink-PS Converter2 : nesl_utility_internal/Simulink-PS Converter  PhysicalDomain=network_engine_domain  SubClassName=ps_input  LeftPortType=input  RightPortType=output  PseudoPeriodic=off  Frequencies=[]  NoiseDistribution=none  NoiseParameters=[]  Unit=1  AffineConversion=off  FilteringAndDerivatives=provide  SimscapeFilterOrder=1  InputFilterTimeConstant=0.001  UdotUserProvided=0
  Vin : fl_lib/Electrical/Electrical Sources/DC Voltage Source  v0=Vin V
  Voltage Sensing : Subsystem
      settings: PortSchema="{\"entries\":[{\"content\":{\"sides\":[{\"content\":{\"connectorIds\":[\"LConn1\"]},\"type\":\"ConnectorPlacement.EquallySpacedRectSide\",\"uuid\":\"8998040f-d19b-40f6-852f-9dc0afd5a871\"},{\"content\":{\"connectorIds\":[\"RConn1\"],\"side\":\"RIGHT\"},\"type\":\"ConnectorPlacement.EquallySpacedRectSide\",\"uuid\":\"65494d6e-d653-4050-90f0-55ab431a5ea5\"},{\"content\":{\"connectorIds\":[],\"side\":\"TOP\"},\"type\":\"ConnectorPlacement.EquallySpacedRectSide\",\"uuid\":\"2b796c8d-afa9-4f67-a302-9fd74e5c5a87\"},{\"content\":{\"connectorIds\":[\"Out1\"],\"side\":\"BOTTOM\"},\"type\":\"ConnectorPlacement.EquallySpacedRectSide\",\"uuid\":\"603bcbba-3a86-43b0-b8d3-5ff10845ef5f\"}]},\"type\":\"ConnectorPlacement.EquallySpacedConnector\",\"uuid\":\"55bdfac7-fde1-4547-95b0-f675ec2b07db\"}],\"packageUris\":[\"http://schema.mathworks.com/mf0/Connector/R2020b\"],\"version\":\"1.0\"}"
      mask Display:
      | disp('V')
      | port_label('Lconn',1,'+')
      | port_label('Rconn',1,'-')
  Voltage Sensing1 : Subsystem
      mask Display:
      | disp('V')
      | port_label('Lconn',1,'+')
      | port_label('Rconn',1,'-')
  Conn1 : PMIOPort  Side=Right
  Conn2 : PMIOPort  Port=2  Side=Right
  Vt : Outport
  It : Outport  Port=2
  Vout : Outport  Port=3
  IL : Outport  Port=4
  wires:
  PID Controller/1(G) -> Simulink-PS Converter2/1
  Voltage Sensing1/1(Vout) -> Scope - DGU 1/1, PID Controller/2(Vout), Vout/1  "Vout_1"
  Iload Value/1 -> Simulink-PS Converter1/1
  Vref/1 -> PID Controller/1(Vref)
  Sensing I/1(Iout) -> Scope - DGU 1/2, It/1  "It_1"
  Voltage Sensing/1(Out1) -> Vt/1
  Sensing I1/1(Iout) -> IL/1
  connections:
  Capacitor1/LConn1 -- Inductor/RConn1 -- Conn1/RConn1 -- Voltage Sensing1/LConn1 -- Controlled Current Source/RConn2
  Vin/LConn1 -- Sensing Vin/LConn1 -- R/LConn1
  Resistor/RConn1 -- Inductor/LConn1
  Voltage Sensing/LConn1 -- Sensing I/RConn1 -- Resistor/LConn1
  Controlled Current Source/RConn1 -- Simulink-PS Converter1/RConn1
  Sensing I1/LConn1 -- Controlled Current Source/LConn1
  Vin/RConn1 -- Average-Value DC-DC Converter/LConn3 -- Sensing Vin/RConn1 -- Electrical Reference1/LConn1
  Capacitor1/RConn1 -- Average-Value DC-DC Converter/RConn2 -- Voltage Sensing/RConn1 -- Voltage Sensing1/RConn1 -- Conn2/RConn1 -- Sensing I1/RConn1
  Average-Value DC-DC Converter/LConn1 -- Simulink-PS Converter2/RConn1
  Average-Value DC-DC Converter/LConn2 -- R/RConn1
  Average-Value DC-DC Converter/RConn1 -- Sensing I/LConn1

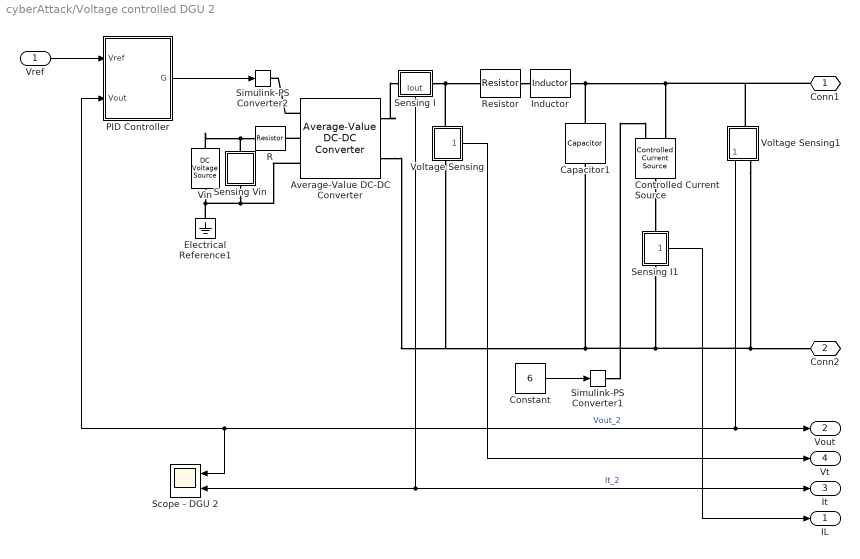
== system cyberAttack/Voltage controlled DGU 2 ==
  Vref : Inport
  Average-Value DC-DC Converter : ee_lib/Semiconductors & Converters/Converters/Average-Value DC-DC Converter  control_option=ee.enum.converters.controlinput.dutycycle  converter_type=ee.enum.converters.dcdctype.buck  efficiency_option=ee.enum.converters.efficiency.constant  efficiency_fixed=100  i_vec=[0, 2, 5] A  efficiency_vec=[90, 95, 98]
      settings: InternalSimscapePortConfiguration="{\"Bottom\":[],\"Left\":[{\"id\":\"DutyCycle\",\"label\":\"DutyCycle\",\"type\":\"input\"},{\"id\":\"p1\",\"label\":\"1+\",\"type\":\"foundation.electrical.electrical\"},{\"id\":\"n1\",\"label\":\"1-\",\"type\":\"foundation.electrical.electrical\"}],\"Right\":[{\"id\":\"p2\",\"label\":\"2+\",\"type\":\"foundation.electrical.electrical\"},{\"id\":\"n2\",\"label\":\"2-\",\"type\":\"foundation.electrical.electrical\"}],\"Top\":[]}"
  Capacitor1 : fl_lib/Electrical/Electrical Elements/Capacitor  c=Ct F  r=1e-6 Ohm  g=0 1/Ohm  i_specify=off  i_priority=None  i=0 A  i_nominal_specify=off  i_nominal_unit=A  i_nominal_value=1  v_specify=on  v_priority=None  v=80 V  v_nominal_specify=off  v_nominal_unit=V  v_nominal_value=1  vc_specify=off  vc_priority=High  vc=0 V  vc_nominal_specify=off  vc_nominal_unit=V  vc_nominal_value=1
  Constant : Constant  Value=6  SampleTime=Ts
  Controlled Current Source : fl_lib/Electrical/Electrical Sources/Controlled Current Source
  Electrical Reference1 : fl_lib/Electrical/Electrical Elements/Electrical Reference
  Inductor : fl_lib/Electrical/Electrical Elements/Inductor  l=Lt H  r=0 Ohm  g=1e-9 1/Ohm  i_specify=off  i_priority=None  i=0 A  i_nominal_specify=off  i_nominal_unit=A  i_nominal_value=1  v_specify=off  v_priority=None  v=0 V  v_nominal_specify=off  v_nominal_unit=V  v_nominal_value=1  i_L_specify=off  i_L_priority=High  i_L=0 A  i_L_nominal_specify=off  i_L_nominal_unit=A  i_L_nominal_value=1
  PID Controller : Subsystem  VariantControl=PID Controller
  R : fl_lib/Electrical/Electrical Elements/Resistor  R=0.001 Ohm  i_specify=off  i_priority=None  i=0 A  i_nominal_specify=off  i_nominal_unit=A  i_nominal_value=1  v_specify=off  v_priority=None  v=0 V  v_nominal_specify=off  v_nominal_unit=V  v_nominal_value=1
  Resistor : fl_lib/Electrical/Electrical Elements/Resistor  R=Rt Ohm  i_specify=off  i_priority=None  i=0 A  i_nominal_specify=off  i_nominal_unit=A  i_nominal_value=1  v_specify=off  v_priority=None  v=0 V  v_nominal_specify=off  v_nominal_unit=V  v_nominal_value=1
  Scope - DGU 2 : Scope  NumInputPorts=2
  Sensing Vin : Subsystem
      mask Display:
      | disp('V')
      | port_label('Lconn',1,'+')
      | port_label('Rconn',1,'-')
  Sensing I : Subsystem
      settings: PortSchema="{\"entries\":[{\"content\":{\"sides\":[{\"content\":{\"connectorIds\":[\"LConn1\"]},\"type\":\"ConnectorPlacement.EquallySpacedRectSide\",\"uuid\":\"8998040f-d19b-40f6-852f-9dc0afd5a871\"},{\"content\":{\"connectorIds\":[\"RConn1\"],\"side\":\"RIGHT\"},\"type\":\"ConnectorPlacement.EquallySpacedRectSide\",\"uuid\":\"65494d6e-d653-4050-90f0-55ab431a5ea5\"},{\"content\":{\"connectorIds\":[],\"side\":\"TOP\"},\"type\":\"ConnectorPlacement.EquallySpacedRectSide\",\"uuid\":\"2b796c8d-afa9-4f67-a302-9fd74e5c5a87\"},{\"content\":{\"connectorIds\":[\"Out1\"],\"side\":\"BOTTOM\"},\"type\":\"ConnectorPlacement.EquallySpacedRectSide\",\"uuid\":\"a59db07b-fad7-4423-9f0d-248c8e243318\"}]},\"type\":\"ConnectorPlacement.EquallySpacedConnector\",\"uuid\":\"55bdfac7-fde1-4547-95b0-f675ec2b07db\"}],\"packageUris\":[\"http://schema.mathworks.com/mf0/Connector/R2020b\"],\"version\":\"1.0\"}"
      mask Display:
      | disp('I')
      | port_label('Lconn',1,'+')
      | port_label('Rconn',1,'-')
  Sensing I1 : Subsystem
      settings: PortSchema="{\"entries\":[{\"content\":{\"sides\":[{\"content\":{\"connectorIds\":[\"LConn1\"]},\"type\":\"ConnectorPlacement.EquallySpacedRectSide\",\"uuid\":\"8998040f-d19b-40f6-852f-9dc0afd5a871\"},{\"content\":{\"connectorIds\":[\"RConn1\"],\"side\":\"RIGHT\"},\"type\":\"ConnectorPlacement.EquallySpacedRectSide\",\"uuid\":\"65494d6e-d653-4050-90f0-55ab431a5ea5\"},{\"content\":{\"connectorIds\":[\"Out1\"],\"side\":\"TOP\"},\"type\":\"ConnectorPlacement.EquallySpacedRectSide\",\"uuid\":\"2b796c8d-afa9-4f67-a302-9fd74e5c5a87\"},{\"content\":{\"connectorIds\":[],\"side\":\"BOTTOM\"},\"type\":\"ConnectorPlacement.EquallySpacedRectSide\",\"uuid\":\"a59db07b-fad7-4423-9f0d-248c8e243318\"}]},\"type\":\"ConnectorPlacement.EquallySpacedConnector\",\"uuid\":\"55bdfac7-fde1-4547-95b0-f675ec2b07db\"}],\"packageUris\":[\"http://schema.mathworks.com/mf0/Connector/R2020b\"],\"version\":\"1.0\"}"
      mask Display:
      | disp('I')
      | port_label('Lconn',1,'+')
      | port_label('Rconn',1,'-')
  Simulink-PS Converter1 : nesl_utility_internal/Simulink-PS Converter  PhysicalDomain=network_engine_domain  SubClassName=ps_input  LeftPortType=input  RightPortType=output  PseudoPeriodic=off  Frequencies=[]  NoiseDistribution=none  NoiseParameters=[]  Unit=1  AffineConversion=off  FilteringAndDerivatives=zero  SimscapeFilterOrder=1  InputFilterTimeConstant=0.001  UdotUserProvided=0
  Simulink-PS Converter2 : nesl_utility_internal/Simulink-PS Converter  PhysicalDomain=network_engine_domain  SubClassName=ps_input  LeftPortType=input  RightPortType=output  PseudoPeriodic=off  Frequencies=[]  NoiseDistribution=none  NoiseParameters=[]  Unit=1  AffineConversion=off  FilteringAndDerivatives=provide  SimscapeFilterOrder=1  InputFilterTimeConstant=0.001  UdotUserProvided=0
  Vin : fl_lib/Electrical/Electrical Sources/DC Voltage Source  v0=Vin V
  Voltage Sensing : Subsystem
      settings: PortSchema="{\"entries\":[{\"content\":{\"sides\":[{\"content\":{\"connectorIds\":[\"LConn1\"]},\"type\":\"ConnectorPlacement.EquallySpacedRectSide\",\"uuid\":\"8998040f-d19b-40f6-852f-9dc0afd5a871\"},{\"content\":{\"connectorIds\":[\"RConn1\"],\"side\":\"RIGHT\"},\"type\":\"ConnectorPlacement.EquallySpacedRectSide\",\"uuid\":\"65494d6e-d653-4050-90f0-55ab431a5ea5\"},{\"content\":{\"connectorIds\":[],\"side\":\"TOP\"},\"type\":\"ConnectorPlacement.EquallySpacedRectSide\",\"uuid\":\"2b796c8d-afa9-4f67-a302-9fd74e5c5a87\"},{\"content\":{\"connectorIds\":[\"Out1\"],\"side\":\"BOTTOM\"},\"type\":\"ConnectorPlacement.EquallySpacedRectSide\",\"uuid\":\"603bcbba-3a86-43b0-b8d3-5ff10845ef5f\"}]},\"type\":\"ConnectorPlacement.EquallySpacedConnector\",\"uuid\":\"55bdfac7-fde1-4547-95b0-f675ec2b07db\"}],\"packageUris\":[\"http://schema.mathworks.com/mf0/Connector/R2020b\"],\"version\":\"1.0\"}"
      mask Display:
      | disp('V')
      | port_label('Lconn',1,'+')
      | port_label('Rconn',1,'-')
  Voltage Sensing1 : Subsystem
      mask Display:
      | disp('V')
      | port_label('Lconn',1,'+')
      | port_label('Rconn',1,'-')
  Conn1 : PMIOPort  Side=Right
  Conn2 : PMIOPort  Port=2  Side=Right
  IL : Outport
  Vout : Outport  Port=2
  It : Outport  Port=3
  Vt : Outport  Port=4
  wires:
  PID Controller/1(G) -> Simulink-PS Converter2/1
  Voltage Sensing1/1(Vout) -> PID Controller/2(Vout), Scope - DGU 2/1, Vout/1  "Vout_2"
  Constant/1 -> Simulink-PS Converter1/1
  Vref/1 -> PID Controller/1(Vref)
  Sensing I/1(Iout) -> It/1, Scope - DGU 2/2  "It_2"
  Voltage Sensing/1(Out1) -> Vt/1
  Sensing I1/1(Iout) -> IL/1
  connections:
  Voltage Sensing1/RConn1 -- Conn2/RConn1 -- Sensing I1/RConn1 -- Capacitor1/RConn1 -- Average-Value DC-DC Converter/RConn2 -- Voltage Sensing/RConn1
  Capacitor1/LConn1 -- Inductor/RConn1 -- Conn1/RConn1 -- Voltage Sensing1/LConn1 -- Controlled Current Source/RConn2
  Sensing Vin/RConn1 -- Average-Value DC-DC Converter/LConn3 -- Electrical Reference1/LConn1 -- Vin/RConn1
  Vin/LConn1 -- Sensing Vin/LConn1 -- R/LConn1
  Resistor/RConn1 -- Inductor/LConn1
  Average-Value DC-DC Converter/RConn1 -- Sensing I/LConn1
  Average-Value DC-DC Converter/LConn2 -- R/RConn1
  Average-Value DC-DC Converter/LConn1 -- Simulink-PS Converter2/RConn1
  Voltage Sensing/LConn1 -- Sensing I/RConn1 -- Resistor/LConn1
  Simulink-PS Converter1/RConn1 -- Controlled Current Source/RConn1
  Controlled Current Source/LConn1 -- Sensing I1/LConn1

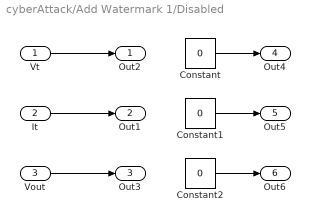
== system cyberAttack/Add Watermark 1/Disabled ==
  Vt : Inport
  It : Inport  Port=2
  Vout : Inport  Port=3
  Constant : Constant  Value=0  SampleTime=Ts
  Constant1 : Constant  Value=0  SampleTime=Ts
  Constant2 : Constant  Value=0  SampleTime=Ts
  Out2 : Outport
  Out1 : Outport  Port=2
  Out3 : Outport  Port=3
  Out4 : Outport  Port=4
  Out5 : Outport  Port=5
  Out6 : Outport  Port=6
  wires:
  Constant2/1 -> Out6/1
  Vout/1 -> Out3/1
  Constant1/1 -> Out5/1
  It/1 -> Out1/1
  Constant/1 -> Out4/1
  Vt/1 -> Out2/1

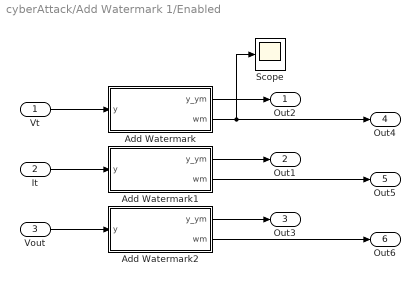
== system cyberAttack/Add Watermark 1/Enabled ==
  Vt : Inport
  It : Inport  Port=2
  Vout : Inport  Port=3
  Add Watermark : Subsystem  mask{MP_SawtoothAmplitude=0.1, MP_SawtoothFrequency=2}
      mask prompts: MP_SawtoothAmplitude "Sawtooth Amplitude"; MP_SawtoothFrequency "Sawtooth Frequency"
      mask DialogControl ParameterGroupVar Prompt: Sawtooth Watermark Signal
  Add Watermark1 : Subsystem  mask{MP_SawtoothAmplitude=0.1, MP_SawtoothFrequency=2}
      mask prompts: MP_SawtoothAmplitude "Sawtooth Amplitude"; MP_SawtoothFrequency "Sawtooth Frequency"
      mask DialogControl ParameterGroupVar Prompt: Sawtooth Watermark Signal
  Add Watermark2 : Subsystem  mask{MP_SawtoothAmplitude=0.1, MP_SawtoothFrequency=2}
      mask prompts: MP_SawtoothAmplitude "Sawtooth Amplitude"; MP_SawtoothFrequency "Sawtooth Frequency"
      mask DialogControl ParameterGroupVar Prompt: Sawtooth Watermark Signal
  Scope : Scope
  Out2 : Outport
  Out1 : Outport  Port=2
  Out3 : Outport  Port=3
  Out4 : Outport  Port=4
  Out5 : Outport  Port=5
  Out6 : Outport  Port=6
  wires:
  Vt/1 -> Add Watermark/1(y)
  It/1 -> Add Watermark1/1(y)
  Vout/1 -> Add Watermark2/1(y)
  Add Watermark/1(y_ym) -> Out2/1
  Add Watermark/2(wm) -> Scope/1, Out4/1
  Add Watermark1/1(y_ym) -> Out1/1
  Add Watermark1/2(wm) -> Out5/1
  Add Watermark2/1(y_ym) -> Out3/1
  Add Watermark2/2(wm) -> Out6/1

== system cyberAttack/Add Watermark 2/Disabled ==
  Vt : Inport
  It : Inport  Port=2
  Vout : Inport  Port=3
  Constant : Constant  Value=0  SampleTime=Ts
  Constant1 : Constant  Value=0  SampleTime=Ts
  Constant2 : Constant  Value=0  SampleTime=Ts
  Out2 : Outport
  Out1 : Outport  Port=2
  Out3 : Outport  Port=3
  Out4 : Outport  Port=4
  Out5 : Outport  Port=5
  Out6 : Outport  Port=6
  wires:
  Constant2/1 -> Out6/1
  Vout/1 -> Out3/1
  Constant1/1 -> Out5/1
  It/1 -> Out1/1
  Constant/1 -> Out4/1
  Vt/1 -> Out2/1

== system cyberAttack/Add Watermark 2/Enabled ==
  Vt : Inport
  It : Inport  Port=2
  Vout : Inport  Port=3
  Add Watermark : Subsystem  mask{MP_SawtoothAmplitude=0.1, MP_SawtoothFrequency=2}
      mask prompts: MP_SawtoothAmplitude "Sawtooth Amplitude"; MP_SawtoothFrequency "Sawtooth Frequency"
      mask DialogControl ParameterGroupVar Prompt: Sawtooth Watermark Signal
  Add Watermark1 : Subsystem  mask{MP_SawtoothAmplitude=0.1, MP_SawtoothFrequency=2}
      mask prompts: MP_SawtoothAmplitude "Sawtooth Amplitude"; MP_SawtoothFrequency "Sawtooth Frequency"
      mask DialogControl ParameterGroupVar Prompt: Sawtooth Watermark Signal
  Add Watermark2 : Subsystem  mask{MP_SawtoothAmplitude=0.1, MP_SawtoothFrequency=2}
      mask prompts: MP_SawtoothAmplitude "Sawtooth Amplitude"; MP_SawtoothFrequency "Sawtooth Frequency"
      mask DialogControl ParameterGroupVar Prompt: Sawtooth Watermark Signal
  Out2 : Outport
  Out1 : Outport  Port=2
  Out3 : Outport  Port=3
  Out4 : Outport  Port=4
  Out5 : Outport  Port=5
  Out6 : Outport  Port=6
  wires:
  Vt/1 -> Add Watermark/1(y)
  It/1 -> Add Watermark1/1(y)
  Vout/1 -> Add Watermark2/1(y)
  Add Watermark/1(y_ym) -> Out2/1
  Add Watermark/2(wm) -> Out4/1
  Add Watermark1/1(y_ym) -> Out1/1
  Add Watermark1/2(wm) -> Out5/1
  Add Watermark2/1(y_ym) -> Out3/1
  Add Watermark2/2(wm) -> Out6/1

== system cyberAttack/Communication Channel DGU 1 (open to attack)/Communication Channel ==
  Vt : Inport
  It : Inport  Port=2
  Vout : Inport  Port=3
  tag scope: It_1=global, Vout_1=global, Vt_1=global
  wires:
  Vout/1 -> [Vout_1]
  It/1 -> [It_1]
  Vt/1 -> [Vt_1]

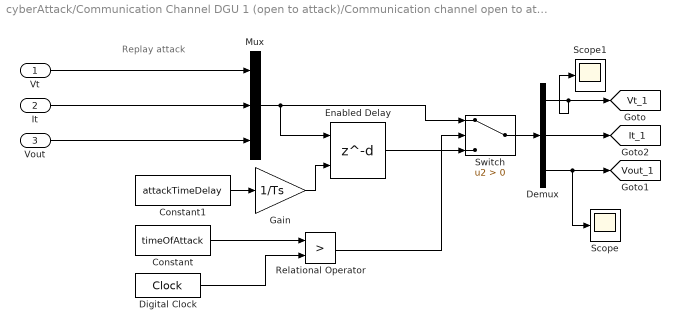
== system cyberAttack/Communication Channel DGU 1 (open to attack)/Communication channel open to attack ==
  note: Replay attack
  Vt : Inport
  It : Inport  Port=2
  Vout : Inport  Port=3
  Constant : Constant  Value=timeOfAttack  SampleTime=1
  Constant1 : Constant  Value=attackTimeDelay
  Demux : Demux  Outputs=3
  Digital Clock : DigitalClock
  Enabled Delay : Delay  DelayLengthSource=Input port  DelayLength=attackTimeDelay/Ts  DelayLengthUpperLimit=4000  SampleTime=Ts
      settings: InputPortMap=u0,p1
  Gain : Gain  Gain=1/Ts
  Mux : Mux  Inputs=3
  Relational Operator : RelationalOperator  Operator=>  OutDataTypeStr=boolean  RndMeth=Simplest  InputSameDT=off
  Scope : Scope
  Scope1 : Scope
  Switch : Switch  Criteria=u2 > Threshold  SaturateOnIntegerOverflow=off  InputSameDT=off
  tag scope: It_1=global, Vout_1=global, Vt_1=global
  wires:
  Demux/1 -> Scope1/1, [Vt_1]
  Demux/2 -> [It_1]
  Demux/3 -> Scope/1, [Vout_1]
  Vout/1 -> Mux/3
  It/1 -> Mux/2
  Vt/1 -> Mux/1
  Constant1/1 -> Gain/1
  Constant/1 -> Relational Operator/1
  Switch/1 -> Demux/1
  Mux/1 -> Switch/1, Enabled Delay/1
  Relational Operator/1 -> Switch/2
  Enabled Delay/1 -> Switch/3
  Digital Clock/1 -> Relational Operator/2
  Gain/1 -> Enabled Delay/2
